simulink model "robot_segway_bloques"  (R2023b)
settings: Solver=ode15s  StartTime=0.0  StopTime=tiempo_final  MaxStep=1e-3  RelTol=1e-5  AbsTol=1e-7
values from neighbouring files (symbols this model uses):
  par = parametros_simulink(P, C)    [cargar_workspace.m]    (also in construir_robot_bloques.m = -R f   (manual sec. 7)'; simular_ode.m)
  Ts = se.Ts    [robot_controlador.m]    (also in simular_ode.m = P.sens.Ts; simular_slx.m = P.sens.Ts)
undefined symbols (not defined in the file or in its folder): angulo_servo_inicial, encoders_iniciales, estados_iniciales, inclinacion_inicial_est, medidas_iniciales, retardo_muestras, semilla
libraries: simulink x10
(part 1 of 2)
settings Model: Creator=calde  LastModifiedBy=calde

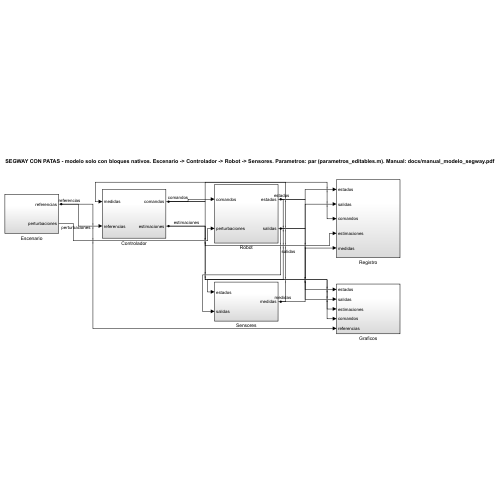
[thumbnail: Simulink's stored preview of the top-level diagram]
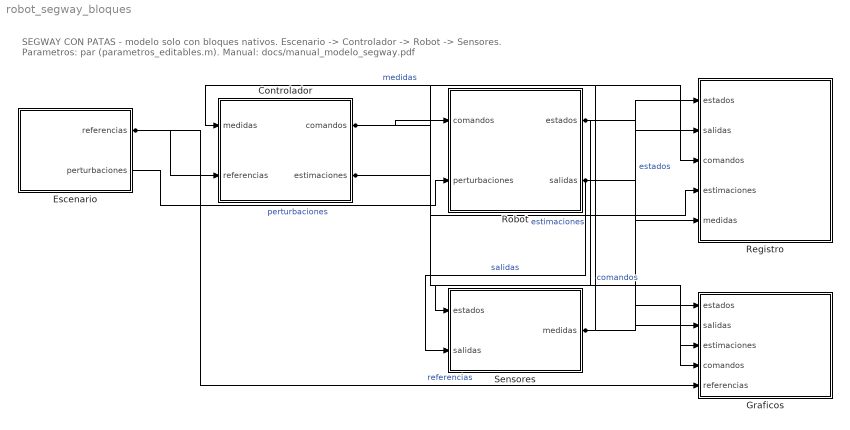
== system robot_segway_bloques ==
  note: SEGWAY CON PATAS - modelo solo con bloques nativos. Escenario -> Controlador -> Robot -> Sensores. Parametros: par (parametros_editables.m). Manual: docs/manual_modelo_segway.pdf
  Controlador : Subsystem
  Escenario : Subsystem
  Graficos : Subsystem
  Registro : Subsystem
  Robot : Subsystem
  Sensores : Subsystem
  wires:
  Escenario/1(referencias) -> Controlador/2(referencias), Graficos/5(referencias)  "referencias"
  Escenario/2(perturbaciones) -> Robot/2(perturbaciones)  "perturbaciones"
  Controlador/1(comandos) -> Robot/1(comandos), Registro/3(comandos), Graficos/4(comandos)  "comandos"
  Robot/1(estados) -> Sensores/1(estados), Registro/1(estados), Graficos/1(estados)  "estados"
  Robot/2(salidas) -> Sensores/2(salidas), Registro/2(salidas), Graficos/2(salidas)  "salidas"
  Sensores/1(medidas) -> Controlador/1(medidas), Registro/5(medidas)  "medidas"
  Controlador/2(estimaciones) -> Registro/4(estimaciones), Graficos/3(estimaciones)  "estimaciones"

== system robot_segway_bloques/Controlador ==
  note: CONTROL discreto a Ts: odometria -> filtro complementario -> LQR programado por l -> tension por motor ; consigna del servo con limite de velocidad
  medidas : Inport
  referencias : Inport  Port=2
  Consigna del servo : Subsystem
  Inclinacion (filtro complementario) : Subsystem
  LQR programado por largo de pata : Subsystem
  Odometria (encoders) : Subsystem
  Par de rueda a tension de motores : Subsystem
  comandos (3) : Mux  Inputs=3
  estimaciones (7) : Mux  Inputs=7
  separar medidas : Demux  Outputs=5
  separar referencias : Demux  Outputs=2
  comandos : Outport
  estimaciones : Outport  Port=2
  wires:
  medidas/1 -> separar medidas/1
  referencias/1 -> separar referencias/1
  separar medidas/4 -> Odometria (encoders)/1(encoder_izq)  "encoder_izq"
  separar medidas/5 -> Odometria (encoders)/2(encoder_der)  "encoder_der"
  separar medidas/1 -> Inclinacion (filtro complementario)/1(giroscopo), LQR programado por largo de pata/5(giroscopo)  "giroscopo"
  separar medidas/2 -> Inclinacion (filtro complementario)/2(acel_x)  "acel_x"
  separar medidas/3 -> Inclinacion (filtro complementario)/3(acel_y)  "acel_y"
  Odometria (encoders)/3(acel_est) -> Inclinacion (filtro complementario)/4(acel_base_est)  "acel_base_est"
  Odometria (encoders)/1(x_est) -> LQR programado por largo de pata/1(x_est), estimaciones (7)/2  "x_est"
  separar referencias/1 -> LQR programado por largo de pata/2(x_ref)  "x_ref"
  Inclinacion (filtro complementario)/1(inclinacion_est) -> LQR programado por largo de pata/3(inclinacion_est), estimaciones (7)/1  "inclinacion_est"
  Odometria (encoders)/2(dx_est) -> LQR programado por largo de pata/4(dx_est), estimaciones (7)/3  "dx_est"
  Consigna del servo/2(angulo_servo_anterior) -> LQR programado por largo de pata/6(angulo_servo_anterior)  "angulo_servo_anterior"
  LQR programado por largo de pata/1(par_rueda) -> Par de rueda a tension de motores/1(par_rueda), estimaciones (7)/5  "par_rueda_cmd"
  Odometria (encoders)/4(vel_ruedas_est) -> Par de rueda a tension de motores/2(vel_ruedas_est)  "vel_ruedas_est"
  separar referencias/2 -> Consigna del servo/1(l_ref)  "l_ref"
  Par de rueda a tension de motores/1(tension_izq) -> comandos (3)/1  "tension_izq"
  Par de rueda a tension de motores/2(tension_der) -> comandos (3)/2  "tension_der"
  Consigna del servo/1(angulo_servo_ref) -> comandos (3)/3  "angulo_servo_ref"
  LQR programado por largo de pata/2(largo_pata_est) -> estimaciones (7)/4  "largo_pata_est"
  Par de rueda a tension de motores/3(saturado) -> estimaciones (7)/6  "tension_saturada"
  Inclinacion (filtro complementario)/2(en_vuelo) -> estimaciones (7)/7  "en_vuelo"
  comandos (3)/1 -> comandos/1
  estimaciones (7)/1 -> estimaciones/1

== system robot_segway_bloques/Escenario ==
  note: Referencias y perturbaciones del escenario (escenarios_robot.m), desde el workspace
  "perturbaciones (F_x, M_p, pendiente, mu, F_escalon)" : FromWorkspace  VariableName=perturbaciones_ts  Interpolate=off  OutputAfterFinalValue=Holding final value
  "referencias (x_ref, l_ref)" : FromWorkspace  VariableName=referencias_ts  SampleTime=Ts  Interpolate=off  OutputAfterFinalValue=Holding final value
  referencias : Outport
  perturbaciones : Outport  Port=2
  wires:
  "referencias (x_ref, l_ref)"/1 -> referencias/1  "referencias"
  "perturbaciones (F_x, M_p, pendiente, mu, F_escalon)"/1 -> perturbaciones/1  "perturbaciones"

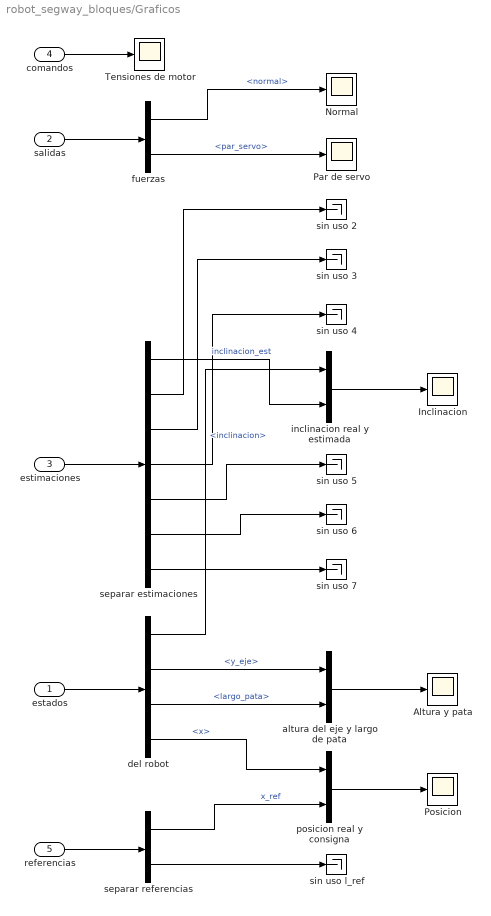
== system robot_segway_bloques/Graficos ==
  estados : Inport
  salidas : Inport  Port=2
  estimaciones : Inport  Port=3
  comandos : Inport  Port=4
  referencias : Inport  Port=5
  Altura y pata : Scope
  Inclinacion : Scope
  Normal : Scope
  Par de servo : Scope
  Posicion : Scope
  Tensiones de motor : Scope
  altura del eje y largo de pata : Mux  Inputs=2
  del robot : BusSelector  OutputSignals=inclinacion,y_eje,largo_pata,x
  fuerzas : BusSelector  OutputSignals=normal,par_servo
  inclinacion real y estimada : Mux  Inputs=2
  posicion real y consigna : Mux  Inputs=2
  separar estimaciones : Demux  Outputs=7
  separar referencias : Demux  Outputs=2
  sin uso {2..7} (6 alike) : Terminator
  sin uso l_ref : Terminator
  wires:
  separar estimaciones/1 -> inclinacion real y estimada/2  "inclinacion_est"
  fuerzas/2 -> Par de servo/1  "<par_servo>"
  comandos/1 -> Tensiones de motor/1
  separar referencias/2 -> sin uso l_ref/1
  salidas/1 -> fuerzas/1
  estimaciones/1 -> separar estimaciones/1
  fuerzas/1 -> Normal/1  "<normal>"
  referencias/1 -> separar referencias/1
  estados/1 -> del robot/1
  separar estimaciones/2 -> sin uso 2/1
  separar estimaciones/3 -> sin uso 3/1
  separar estimaciones/4 -> sin uso 4/1
  separar estimaciones/5 -> sin uso 5/1
  separar estimaciones/6 -> sin uso 6/1
  separar estimaciones/7 -> sin uso 7/1
  del robot/1 -> inclinacion real y estimada/1  "<inclinacion>"
  altura del eje y largo de pata/1 -> Altura y pata/1
  del robot/2 -> altura del eje y largo de pata/1  "<y_eje>"
  del robot/3 -> altura del eje y largo de pata/2  "<largo_pata>"
  del robot/4 -> posicion real y consigna/1  "<x>"
  separar referencias/1 -> posicion real y consigna/2  "x_ref"
  inclinacion real y estimada/1 -> Inclinacion/1
  posicion real y consigna/1 -> Posicion/1

== system robot_segway_bloques/Registro ==
  note: Se guardan en el workspace: estados, salidas, comandos, estimaciones, medidas (simular_slx los convierte en matrices)
  estados : Inport
  salidas : Inport  Port=2
  comandos : Inport  Port=3
  estimaciones : Inport  Port=4
  medidas : Inport  Port=5
  a workspace: comandos : ToWorkspace  VariableName=comandos  SaveFormat=Timeseries  SampleTime=-1
  a workspace: estados : ToWorkspace  VariableName=estados  SaveFormat=Timeseries  SampleTime=-1
  a workspace: estimaciones : ToWorkspace  VariableName=estimaciones  SaveFormat=Timeseries  SampleTime=-1
  a workspace: medidas : ToWorkspace  VariableName=medidas  SaveFormat=Timeseries  SampleTime=-1
  a workspace: salidas : ToWorkspace  VariableName=salidas  SaveFormat=Timeseries  SampleTime=-1
  wires:
  estimaciones/1 -> a workspace: estimaciones/1
  salidas/1 -> a workspace: salidas/1
  medidas/1 -> a workspace: medidas/1
  comandos/1 -> a workspace: comandos/1
  estados/1 -> a workspace: estados/1

== system robot_segway_bloques/Robot ==
  note: PLANTA: cada parte publica un bus con su nombre y los demas eligen lo que usan (Bus Selector). Estados y salidas en el mismo orden que robot_planta.m
  comandos : Inport
  perturbaciones : Inport  Port=2
  Bateria y puente H : Subsystem
  Contacto rueda-piso : Subsystem
  Cuerpo (Lagrange) : Subsystem
  Estados y salidas con nombre : Subsystem
  IMU (fuerza especifica) : Subsystem
  Motores y reductores : Subsystem
  Piso con escalones : Subsystem
  Ruedas : Subsystem
  Servo y pata : Subsystem
  bus comandos : BusCreator  Inputs=3
  bus perturbaciones : BusCreator  Inputs=5
  separar comandos : Demux  Outputs=3
  separar perturbaciones : Demux  Outputs=5
  estados : Outport
  salidas : Outport  Port=2
  wires:
  comandos/1 -> separar comandos/1
  separar comandos/1 -> bus comandos/1  "tension_izq"
  separar comandos/2 -> bus comandos/2  "tension_der"
  separar comandos/3 -> bus comandos/3  "angulo_servo_ref"
  perturbaciones/1 -> separar perturbaciones/1
  separar perturbaciones/1 -> bus perturbaciones/1  "F_x"
  separar perturbaciones/2 -> bus perturbaciones/2  "M_p"
  separar perturbaciones/3 -> bus perturbaciones/3  "pendiente"
  separar perturbaciones/4 -> bus perturbaciones/4  "mu"
  separar perturbaciones/5 -> bus perturbaciones/5  "F_escalon"
  bus comandos/1 -> Bateria y puente H/1(comandos), Servo y pata/1(comandos)  "comandos"
  bus perturbaciones/1 -> Contacto rueda-piso/4(perturbaciones), Cuerpo (Lagrange)/4(perturbaciones), IMU (fuerza especifica)/2(perturbaciones)  "perturbaciones"
  Bateria y puente H/1(bateria) -> Motores y reductores/1(bateria), Estados y salidas con nombre/5(bateria)  "bateria"
  Motores y reductores/1(motores) -> Bateria y puente H/2(motores), Ruedas/1(motores), Cuerpo (Lagrange)/2(motores), Estados y salidas con nombre/3(motores)  "motores"
  Ruedas/1(ruedas) -> Motores y reductores/2(ruedas), Contacto rueda-piso/2(ruedas), Estados y salidas con nombre/2(ruedas)  "ruedas"
  Piso con escalones/1(piso) -> Contacto rueda-piso/3(piso), Estados y salidas con nombre/7(piso)  "piso"
  Contacto rueda-piso/1(contacto) -> Ruedas/2(contacto), Cuerpo (Lagrange)/1(contacto), Estados y salidas con nombre/6(contacto)  "contacto"
  Servo y pata/1(pata) -> Cuerpo (Lagrange)/3(pata), Estados y salidas con nombre/4(pata)  "pata"
  Cuerpo (Lagrange)/1(cuerpo) -> Piso con escalones/1(cuerpo), Contacto rueda-piso/1(cuerpo), Servo y pata/2(cuerpo), IMU (fuerza especifica)/1(cuerpo), Estados y salidas con nombre/1(cuerpo)  "cuerpo"
  IMU (fuerza especifica)/1(imu) -> Estados y salidas con nombre/8(imu)  "imu"
  Estados y salidas con nombre/1(estados) -> estados/1  "estados"
  Estados y salidas con nombre/2(salidas) -> salidas/1  "salidas"

== system robot_segway_bloques/Sensores ==
  note: IMU y encoders muestreados a Ts: giroscopo con sesgo, ruido y saturacion ; acelerometro con ruido ; encoders en cuentas enteras ; retardo de retardo_muestras
  estados : Inport
  salidas : Inport  Port=2
  Acelerometro : Subsystem
  Encoders : Subsystem
  Giroscopio : Subsystem
  de la IMU : BusSelector  OutputSignals=imu_fx,imu_fy
  del robot : BusSelector  OutputSignals=d_inclinacion,ang_rueda_izq,ang_rueda_der
  medidas (5) : Mux  Inputs=5
  muestreo del giro : ZeroOrderHold  SampleTime=Ts
  muestreo f_x : ZeroOrderHold  SampleTime=Ts
  muestreo f_y : ZeroOrderHold  SampleTime=Ts
  muestreo rueda der : ZeroOrderHold  SampleTime=Ts
  muestreo rueda izq : ZeroOrderHold  SampleTime=Ts
  retardo del bus de sensores : Delay  DelayLength=retardo_muestras  InitialCondition=medidas_iniciales  SampleTime=Ts
  medidas : Outport
  wires:
  del robot/3 -> muestreo rueda der/1  "<ang_rueda_der>"
  Encoders/2(encoder_der) -> medidas (5)/5  "encoder_der"
  de la IMU/2 -> muestreo f_y/1  "<imu_fy>"
  salidas/1 -> de la IMU/1
  estados/1 -> del robot/1
  muestreo del giro/1 -> Giroscopio/1(vel_cabeceo)  "vel_cabeceo"
  del robot/2 -> muestreo rueda izq/1  "<ang_rueda_izq>"
  Acelerometro/2(acel_y) -> medidas (5)/3  "acel_y"
  de la IMU/1 -> muestreo f_x/1  "<imu_fx>"
  del robot/1 -> muestreo del giro/1  "<d_inclinacion>"
  muestreo f_x/1 -> Acelerometro/1(f_x)  "f_x"
  Encoders/1(encoder_izq) -> medidas (5)/4  "encoder_izq"
  muestreo f_y/1 -> Acelerometro/2(f_y)  "f_y"
  medidas (5)/1 -> retardo del bus de sensores/1  "medidas_sin_retardo"
  muestreo rueda izq/1 -> Encoders/1(ang_izq)  "ang_izq"
  muestreo rueda der/1 -> Encoders/2(ang_der)  "ang_der"
  Giroscopio/1(giroscopo) -> medidas (5)/1  "giroscopo"
  Acelerometro/1(acel_x) -> medidas (5)/2  "acel_x"
  retardo del bus de sensores/1 -> medidas/1  "medidas"

== system robot_segway_bloques/Controlador/Consigna del servo ==
  note: theta_ref = theta(l_ref) con limite de velocidad 0.8 w_vacio y acotada al rango del servo
  l_ref : Inport
  angulo objetivo theta(l_ref) : Lookup_n-D  NumberOfTableDimensions=1  BreakpointsForDimension1=par.pata.tabla_l  Table=par.pata.tabla_theta  InternalRulePriority=Speed  RndMeth=Simplest
  consigna anterior : UnitDelay  InitialCondition=angulo_servo_inicial  SampleTime=Ts  HasFrameUpgradeWarning=on
  largo dentro de la carrera : Saturate  UpperLimit=par.pata.l_max  LowerLimit=par.pata.l_min
  limitador de velocidad del servo : RateLimiter  RisingSlewLimit=0.8*par.servo.w_vacio  FallingSlewLimit=-(0.8*par.servo.w_vacio)  SampleTimeMode=inherited  InitialCondition=angulo_servo_inicial
  rango del servo : Saturate  UpperLimit=par.servo.theta_max  LowerLimit=par.servo.theta_min
  angulo_servo_ref : Outport
  angulo_servo_anterior : Outport  Port=2
  wires:
  consigna anterior/1 -> angulo_servo_anterior/1
  limitador de velocidad del servo/1 -> rango del servo/1
  l_ref/1 -> largo dentro de la carrera/1
  rango del servo/1 -> consigna anterior/1, angulo_servo_ref/1  "angulo_servo_ref"
  angulo objetivo theta(l_ref)/1 -> limitador de velocidad del servo/1  "angulo_objetivo"
  largo dentro de la carrera/1 -> angulo objetivo theta(l_ref)/1  "l_ref_acotado"

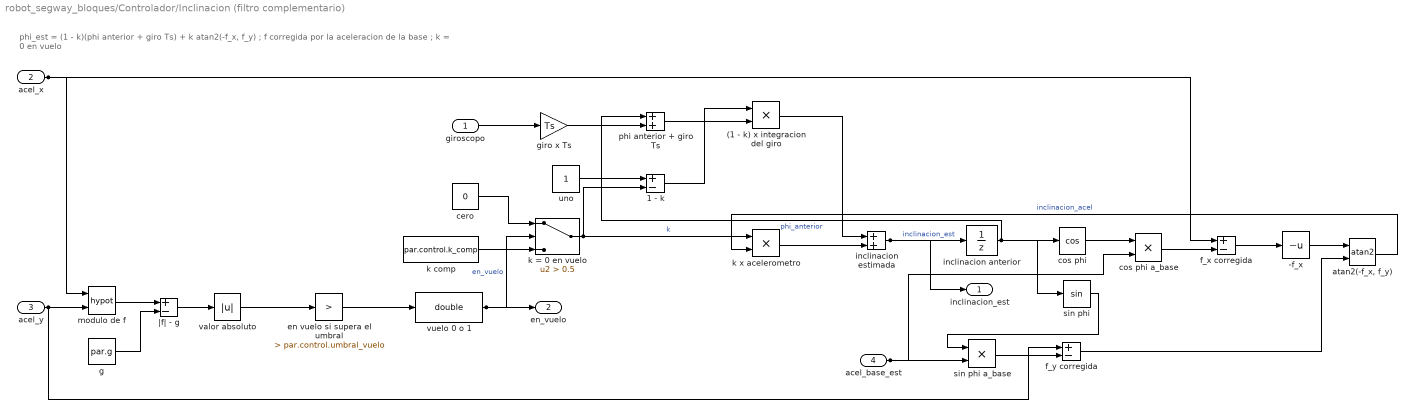
== system robot_segway_bloques/Controlador/Inclinacion (filtro complementario) ==
  note: phi_est = (1 - k)(phi anterior + giro Ts) + k atan2(-f_x, f_y) ; f corregida por la aceleracion de la base ; k = 0 en vuelo
  giroscopo : Inport
  acel_x : Inport  Port=2
  acel_y : Inport  Port=3
  acel_base_est : Inport  Port=4
  (1 - k) x integracion del giro : Product  Inputs=**
  -f_x : UnaryMinus
  1 - k : Sum  Inputs=+-
  "atan2(-f_x, f_y)" : Trigonometry  Operator=atan2
  cero : Constant  Value=0
  cos phi : Trigonometry  Operator=cos
  cos phi a_base : Product  Inputs=**
  en vuelo si supera el umbral : simulink/Logic and Bit Operations/Compare To Constant  relop=>  const=par.control.umbral_vuelo  OutDataTypeStr=boolean
  f_x corregida : Sum  Inputs=+-
  f_y corregida : Sum  Inputs=+-
  g : Constant  Value=par.g
  giro x Ts : Gain  Gain=Ts
  inclinacion anterior : UnitDelay  InitialCondition=inclinacion_inicial_est  SampleTime=Ts  HasFrameUpgradeWarning=on
  inclinacion estimada : Sum
  k = 0 en vuelo : Switch  Criteria=u2 > Threshold  Threshold=0.5  SaturateOnIntegerOverflow=off  InputSameDT=off
  k comp : Constant  Value=par.control.k_comp
  k x acelerometro : Product  Inputs=**
  modulo de f : Math  Operator=hypot
  phi anterior + giro Ts : Sum
  sin phi : Trigonometry
  sin phi a_base : Product  Inputs=**
  uno : Constant
  valor absoluto : Abs  SaturateOnIntegerOverflow=off
  vuelo 0 o 1 : DataTypeConversion  OutDataTypeStr=double  SaturateOnIntegerOverflow=off  RndMeth=Floor
  |f| - g : Sum  Inputs=+-
  inclinacion_est : Outport
  en_vuelo : Outport  Port=2
  wires:
  giroscopo/1 -> giro x Ts/1
  acel_y/1 -> f_y corregida/1, modulo de f/2
  acel_base_est/1 -> cos phi a_base/2, sin phi a_base/2
  (1 - k) x integracion del giro/1 -> inclinacion estimada/1
  acel_x/1 -> f_x corregida/1, modulo de f/1
  1 - k/1 -> (1 - k) x integracion del giro/1
  modulo de f/1 -> |f| - g/1
  g/1 -> |f| - g/2
  |f| - g/1 -> valor absoluto/1
  valor absoluto/1 -> en vuelo si supera el umbral/1
  en vuelo si supera el umbral/1 -> vuelo 0 o 1/1
  phi anterior + giro Ts/1 -> (1 - k) x integracion del giro/2
  cero/1 -> k = 0 en vuelo/1
  -f_x/1 -> "atan2(-f_x, f_y)"/1
  k comp/1 -> k = 0 en vuelo/3
  vuelo 0 o 1/1 -> en_vuelo/1, k = 0 en vuelo/2  "en_vuelo"
  giro x Ts/1 -> phi anterior + giro Ts/2
  uno/1 -> 1 - k/1
  k = 0 en vuelo/1 -> k x acelerometro/1, 1 - k/2  "k"
  k x acelerometro/1 -> inclinacion estimada/2
  "atan2(-f_x, f_y)"/1 -> k x acelerometro/2  "inclinacion_acel"
  inclinacion estimada/1 -> inclinacion anterior/1, inclinacion_est/1  "inclinacion_est"
  inclinacion anterior/1 -> phi anterior + giro Ts/1, sin phi/1, cos phi/1  "phi_anterior"
  cos phi a_base/1 -> f_x corregida/2
  sin phi a_base/1 -> f_y corregida/2
  sin phi/1 -> sin phi a_base/1
  cos phi/1 -> cos phi a_base/1
  f_y corregida/1 -> "atan2(-f_x, f_y)"/2
  f_x corregida/1 -> -f_x/1

== system robot_segway_bloques/Controlador/LQR programado por largo de pata ==
  note: par de rueda = -K(l) [x - x_ref ; phi ; dx ; dphi], K(l) = K1 + K2 l (manual sec. 10)
  x_est : Inport
  x_ref : Inport  Port=2
  inclinacion_est : Inport  Port=3
  dx_est : Inport  Port=4
  giroscopo : Inport  Port=5
  angulo_servo_anterior : Inport  Port=6
  K . error : DotProduct  OutDataTypeStr=Inherit: Inherit via internal rule
  K(l) = K1 + K2 l : Sum
  K1 : Constant  Value=par.control.K1(:)
  K2 x l : Gain  Gain=par.control.K2(:)
  dentro del rango del ajuste : Saturate  UpperLimit=par.control.l_max  LowerLimit=par.control.l_min
  error = [x - x_ref; phi; dx; dphi] : Mux
  error de posicion : Sum  Inputs=+-
  largo de pata segun angulo del servo : Lookup_n-D  NumberOfTableDimensions=1  BreakpointsForDimension1=par.pata.tabla_theta_inv  Table=par.pata.tabla_l_inv  InternalRulePriority=Speed  RndMeth=Simplest
  par = -K . error : UnaryMinus
  par_rueda : Outport
  largo_pata_est : Outport  Port=2
  wires:
  dx_est/1 -> error = [x - x_ref; phi; dx; dphi]/3
  angulo_servo_anterior/1 -> largo de pata segun angulo del servo/1
  largo de pata segun angulo del servo/1 -> dentro del rango del ajuste/1, largo_pata_est/1  "largo_pata_est"
  error de posicion/1 -> error = [x - x_ref; phi; dx; dphi]/1
  K2 x l/1 -> K(l) = K1 + K2 l/2
  dentro del rango del ajuste/1 -> K2 x l/1
  x_ref/1 -> error de posicion/2
  x_est/1 -> error de posicion/1
  K1/1 -> K(l) = K1 + K2 l/1
  giroscopo/1 -> error = [x - x_ref; phi; dx; dphi]/4
  inclinacion_est/1 -> error = [x - x_ref; phi; dx; dphi]/2
  K(l) = K1 + K2 l/1 -> K . error/1  "K"
  error = [x - x_ref; phi; dx; dphi]/1 -> K . error/2  "error"
  K . error/1 -> par = -K . error/1
  par = -K . error/1 -> par_rueda/1

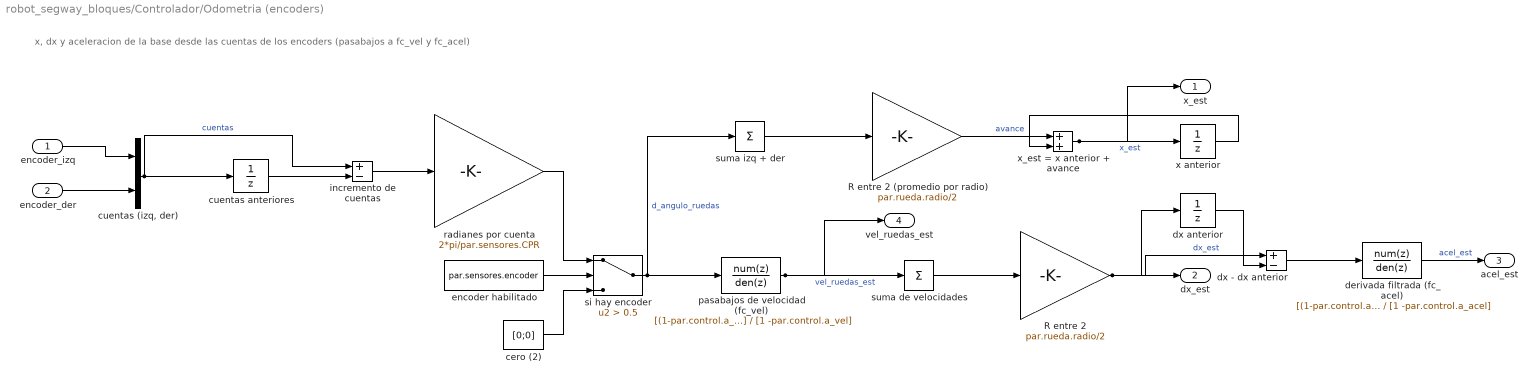
== system robot_segway_bloques/Controlador/Odometria (encoders) ==
  note: x, dx y aceleracion de la base desde las cuentas de los encoders (pasabajos a fc_vel y fc_acel)
  encoder_izq : Inport
  encoder_der : Inport  Port=2
  R entre 2 : Gain  Gain=par.rueda.radio/2
  R entre 2 (promedio por radio) : Gain  Gain=par.rueda.radio/2
  cero (2) : Constant  Value=[0;0]
  "cuentas (izq, der)" : Mux  Inputs=2
  cuentas anteriores : UnitDelay  InitialCondition=encoders_iniciales  SampleTime=Ts  HasFrameUpgradeWarning=on
  derivada filtrada (fc_acel) : DiscreteTransferFcn  Numerator=[(1-par.control.a_acel)/Ts 0]  Denominator=[1 -par.control.a_acel]  SampleTime=Ts
  dx - dx anterior : Sum  Inputs=+-
  dx anterior : UnitDelay  SampleTime=Ts  HasFrameUpgradeWarning=on
  encoder habilitado : Constant  Value=par.sensores.encoder
  incremento de cuentas : Sum  Inputs=+-
  pasabajos de velocidad (fc_vel) : DiscreteTransferFcn  Numerator=[(1-par.control.a_vel)/Ts 0]  Denominator=[1 -par.control.a_vel]  SampleTime=Ts
  radianes por cuenta : Gain  Gain=2*pi/par.sensores.CPR
  si hay encoder : Switch  Criteria=u2 > Threshold  Threshold=0.5  SaturateOnIntegerOverflow=off  InputSameDT=off
  suma de velocidades : Sum  Inputs=+
  suma izq + der : Sum  Inputs=+
  x anterior : UnitDelay  SampleTime=Ts  HasFrameUpgradeWarning=on
  x_est = x anterior + avance : Sum
  x_est : Outport
  dx_est : Outport  Port=2
  acel_est : Outport  Port=3
  vel_ruedas_est : Outport  Port=4
  wires:
  encoder_der/1 -> "cuentas (izq, der)"/2
  radianes por cuenta/1 -> si hay encoder/1
  R entre 2/1 -> dx - dx anterior/1, dx anterior/1, dx_est/1  "dx_est"
  encoder_izq/1 -> "cuentas (izq, der)"/1
  cero (2)/1 -> si hay encoder/3
  "cuentas (izq, der)"/1 -> incremento de cuentas/1, cuentas anteriores/1  "cuentas"
  cuentas anteriores/1 -> incremento de cuentas/2
  derivada filtrada (fc_acel)/1 -> acel_est/1  "acel_est"
  dx - dx anterior/1 -> derivada filtrada (fc_acel)/1
  incremento de cuentas/1 -> radianes por cuenta/1
  encoder habilitado/1 -> si hay encoder/2
  si hay encoder/1 -> pasabajos de velocidad (fc_vel)/1, suma izq + der/1  "d_angulo_ruedas"
  R entre 2 (promedio por radio)/1 -> x_est = x anterior + avance/1  "avance"
  suma izq + der/1 -> R entre 2 (promedio por radio)/1
  x_est = x anterior + avance/1 -> x anterior/1, x_est/1  "x_est"
  pasabajos de velocidad (fc_vel)/1 -> vel_ruedas_est/1, suma de velocidades/1  "vel_ruedas_est"
  dx anterior/1 -> dx - dx anterior/2
  suma de velocidades/1 -> R entre 2/1
  x anterior/1 -> x_est = x anterior + avance/2

== system robot_segway_bloques/Controlador/Par de rueda a tension de motores ==
  note: V = R (tau/2)/(Kt N eta) + Ke N w_est por motor, saturada a +-V_bat
  par_rueda : Inport
  vel_ruedas_est : Inport  Port=2
  R entre (2 Kt N eta) : Gain  Gain=par.motor.R/(2*par.motor.Kt*par.motor.relacion*par.motor.eta)
  alguna satura : Logic  Operator=OR  Inputs=1  AllPortsSameDT=off  OutDataTypeStr=boolean
  fcem Ke N w : Gain  Gain=par.motor.Ke*par.motor.relacion
  izq y der : Demux  Outputs=2
  limitar a la bateria : Saturate  UpperLimit=par.bateria.V  LowerLimit=-par.bateria.V
  saturado 0 o 1 : DataTypeConversion  OutDataTypeStr=double  SaturateOnIntegerOverflow=off  RndMeth=Floor
  supera V_bat : simulink/Logic and Bit Operations/Compare To Constant  relop=>  const=par.bateria.V  OutDataTypeStr=boolean
  "tension pedida (izq, der)" : Sum
  |V| : Abs  SaturateOnIntegerOverflow=off
  tension_izq : Outport
  tension_der : Outport  Port=2
  saturado : Outport  Port=3
  wires:
  par_rueda/1 -> R entre (2 Kt N eta)/1
  fcem Ke N w/1 -> "tension pedida (izq, der)"/2  "por_la_fcem"
  R entre (2 Kt N eta)/1 -> "tension pedida (izq, der)"/1  "por_el_par"
  vel_ruedas_est/1 -> fcem Ke N w/1
  limitar a la bateria/1 -> izq y der/1  "tension"
  "tension pedida (izq, der)"/1 -> |V|/1, limitar a la bateria/1  "tension_pedida"
  |V|/1 -> supera V_bat/1
  izq y der/1 -> tension_izq/1
  izq y der/2 -> tension_der/1
  supera V_bat/1 -> alguna satura/1
  alguna satura/1 -> saturado 0 o 1/1
  saturado 0 o 1/1 -> saturado/1

== system robot_segway_bloques/Robot/Bateria y puente H ==
  note: V_bus = max(V_bat - R_bat (|i_izq| + |i_der|), 0) ; V aplicada = sat(V pedida, -V_bus .. V_bus)
  comandos : Inport
  motores : Inport  Port=2
  -V_bus : UnaryMinus
  V_bat : Constant  Value=par.bateria.V
  V_bat - caida : Sum  Inputs=+-
  bus bateria : BusCreator  Inputs=3
  caida R_bat i : Gain  Gain=par.bateria.R
  cero : Constant  Value=0
  corriente total : Sum
  corrientes : BusSelector  OutputSignals=corriente_izq,corriente_der
  limitar der : simulink/Discontinuities/Saturation Dynamic  OutMin=[]  OutMax=[]  OutDataTypeStr=Inherit: Same as second input  OutDataType=fixdt(1, 16)  OutScaling=2^-10  DoSatur=off
  limitar izq : simulink/Discontinuities/Saturation Dynamic  OutMin=[]  OutMax=[]  OutDataTypeStr=Inherit: Same as second input  OutDataType=fixdt(1, 16)  OutScaling=2^-10  DoSatur=off
  no menor que 0 : MinMax  Function=max  Inputs=2
  tensiones pedidas : BusSelector  OutputSignals=tension_izq,tension_der
  |i der| : Abs  SaturateOnIntegerOverflow=off
  |i izq| : Abs  SaturateOnIntegerOverflow=off
  bateria : Outport
  wires:
  comandos/1 -> tensiones pedidas/1
  V_bat/1 -> V_bat - caida/1
  motores/1 -> corrientes/1
  corrientes/2 -> |i der|/1  "<corriente_der>"
  cero/1 -> no menor que 0/2
  corrientes/1 -> |i izq|/1  "<corriente_izq>"
  |i izq|/1 -> corriente total/1
  |i der|/1 -> corriente total/2
  no menor que 0/1 -> limitar izq/1, limitar der/1, bus bateria/1, -V_bus/1  "tension_bus"
  V_bat - caida/1 -> no menor que 0/1
  caida R_bat i/1 -> V_bat - caida/2  "caida"
  corriente total/1 -> caida R_bat i/1  "corriente_total"
  tensiones pedidas/1 -> limitar izq/2  "<tension_izq>"
  tensiones pedidas/2 -> limitar der/2  "<tension_der>"
  -V_bus/1 -> limitar der/3, limitar izq/3  "-tension_bus"
  limitar izq/1 -> bus bateria/2  "tension_aplicada_izq"
  limitar der/1 -> bus bateria/3  "tension_aplicada_der"
  bus bateria/1 -> bateria/1

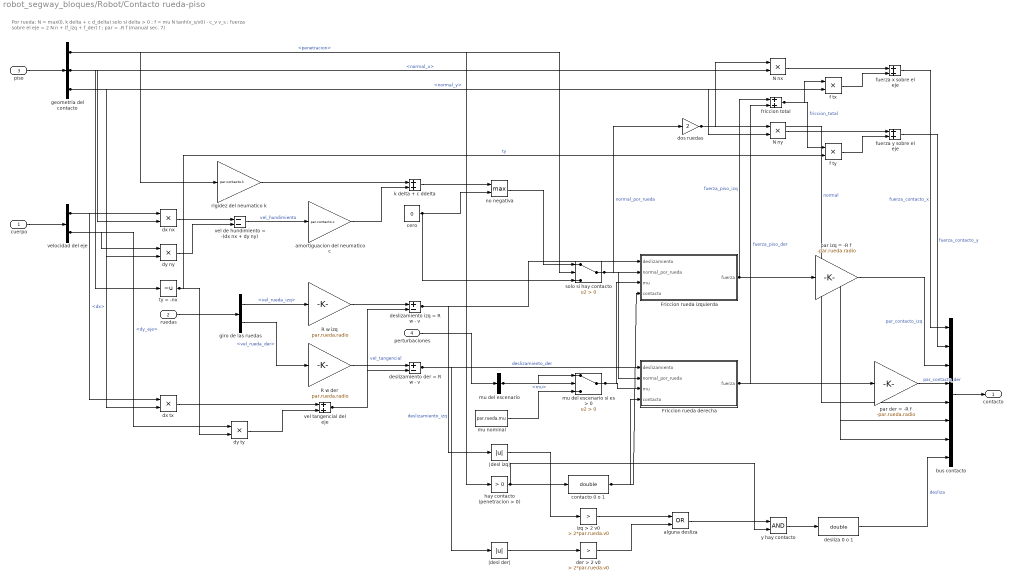
== system robot_segway_bloques/Robot/Contacto rueda-piso ==
  note: Por rueda: N = max(0, k delta + c d_delta) solo si delta > 0 ; f = mu N tanh(v_s/v0) - c_v v_s ; fuerza sobre el eje = 2 N n + (f_izq + f_der) t ; par = -R f (manual sec. 7)
  cuerpo : Inport
  ruedas : Inport  Port=2
  piso : Inport  Port=3
  perturbaciones : Inport  Port=4
  Friccion rueda derecha : Subsystem
  Friccion rueda izquierda : Subsystem
  N nx : Product  Inputs=**
  N ny : Product  Inputs=**
  R w der : Gain  Gain=par.rueda.radio
  R w izq : Gain  Gain=par.rueda.radio
  alguna desliza : Logic  Operator=OR  AllPortsSameDT=off  OutDataTypeStr=boolean
  amortiguacion del neumatico c : Gain  Gain=par.contacto.c
  bus contacto : BusCreator  Inputs=8
  cero : Constant  Value=0
  contacto 0 o 1 : DataTypeConversion  OutDataTypeStr=double  SaturateOnIntegerOverflow=off  RndMeth=Floor
  der > 2 v0 : simulink/Logic and Bit Operations/Compare To Constant  relop=>  const=2*par.rueda.v0  OutDataTypeStr=boolean
  desliza 0 o 1 : DataTypeConversion  OutDataTypeStr=double  SaturateOnIntegerOverflow=off  RndMeth=Floor
  deslizamiento der = R w - v : Sum  Inputs=+-
  deslizamiento izq = R w - v : Sum  Inputs=+-
  dos ruedas : Gain  Gain=2
  dx nx : Product  Inputs=**
  dx tx : Product  Inputs=**
  dy ny : Product  Inputs=**
  dy ty : Product  Inputs=**
  f tx : Product  Inputs=**
  f ty : Product  Inputs=**
  friccion total : Sum
  fuerza x sobre el eje : Sum
  fuerza y sobre el eje : Sum
  geometria del contacto : BusSelector  OutputSignals=penetracion,normal_x,normal_y
  giro de las ruedas : BusSelector  OutputSignals=vel_rueda_izq,vel_rueda_der
  hay contacto (penetracion > 0) : simulink/Logic and Bit Operations/Compare To Zero  relop=>  OutDataTypeStr=boolean
  izq > 2 v0 : simulink/Logic and Bit Operations/Compare To Constant  relop=>  const=2*par.rueda.v0  OutDataTypeStr=boolean
  k delta + c ddelta : Sum
  mu del escenario : BusSelector  OutputSignals=mu
  mu del escenario si es > 0 : Switch  Criteria=u2 > Threshold  SaturateOnIntegerOverflow=off  InputSameDT=off
  mu nominal : Constant  Value=par.rueda.mu
  no negativa : MinMax  Function=max  Inputs=2
  par der = -R f : Gain  Gain=-par.rueda.radio
  par izq = -R f : Gain  Gain=-par.rueda.radio
  rigidez del neumatico k : Gain  Gain=par.contacto.k
  solo si hay contacto : Switch  Criteria=u2 > Threshold  SaturateOnIntegerOverflow=off  InputSameDT=off
  ty = -nx : UnaryMinus
  vel de hundimiento = -(dx nx + dy ny) : Sum  Inputs=--
  vel tangencial del eje : Sum
  velocidad del eje : BusSelector  OutputSignals=dx,dy_eje
  y hay contacto : Logic  AllPortsSameDT=off  OutDataTypeStr=boolean
  |desl der| : Abs  SaturateOnIntegerOverflow=off
  |desl izq| : Abs  SaturateOnIntegerOverflow=off
  contacto : Outport
  wires:
  alguna desliza/1 -> y hay contacto/1
  no negativa/1 -> solo si hay contacto/1
  cuerpo/1 -> velocidad del eje/1
  mu del escenario si es > 0/1 -> Friccion rueda derecha/3(mu), Friccion rueda izquierda/3(mu)
  dx tx/1 -> vel tangencial del eje/1
  piso/1 -> geometria del contacto/1
  velocidad del eje/2 -> dy ty/1, dy ny/1  "<dy_eje>"
  geometria del contacto/3 -> f tx/2, N ny/2, dx tx/2, dy ny/2  "<normal_y>"
  velocidad del eje/1 -> dx nx/1, dx tx/1  "<dx>"
  desliza 0 o 1/1 -> bus contacto/8  "desliza"
  geometria del contacto/2 -> N nx/2, dx nx/2, ty = -nx/1  "<normal_x>"
  geometria del contacto/1 -> hay contacto (penetracion > 0)/1, rigidez del neumatico k/1, solo si hay contacto/2  "<penetracion>"
  solo si hay contacto/1 -> Friccion rueda izquierda/2(normal_por_rueda), Friccion rueda derecha/2(normal_por_rueda), dos ruedas/1  "normal_por_rueda"
  dx nx/1 -> vel de hundimiento = -(dx nx + dy ny)/1
  dy ny/1 -> vel de hundimiento = -(dx nx + dy ny)/2
  ty = -nx/1 -> f ty/2, dy ty/2  "ty"
  cero/1 -> solo si hay contacto/3, no negativa/2
  ruedas/1 -> giro de las ruedas/1
  vel de hundimiento = -(dx nx + dy ny)/1 -> amortiguacion del neumatico c/1  "vel_hundimiento"
  rigidez del neumatico k/1 -> k delta + c ddelta/1
  giro de las ruedas/1 -> R w izq/1  "<vel_rueda_izq>"
  giro de las ruedas/2 -> R w der/1  "<vel_rueda_der>"
  amortiguacion del neumatico c/1 -> k delta + c ddelta/2
  dy ty/1 -> vel tangencial del eje/2
  vel tangencial del eje/1 -> deslizamiento izq = R w - v/2, deslizamiento der = R w - v/2  "vel_tangencial"
  R w izq/1 -> deslizamiento izq = R w - v/1
  R w der/1 -> deslizamiento der = R w - v/1
  k delta + c ddelta/1 -> no negativa/1
  deslizamiento izq = R w - v/1 -> Friccion rueda izquierda/1(deslizamiento), |desl izq|/1  "deslizamiento_izq"
  perturbaciones/1 -> mu del escenario/1
  f tx/1 -> fuerza x sobre el eje/2
  deslizamiento der = R w - v/1 -> Friccion rueda derecha/1(deslizamiento), |desl der|/1  "deslizamiento_der"
  mu del escenario/1 -> mu del escenario si es > 0/1, mu del escenario si es > 0/2  "<mu>"
  Friccion rueda derecha/1(fuerza) -> par der = -R f/1, friccion total/2, bus contacto/7  "fuerza_piso_der"
  mu nominal/1 -> mu del escenario si es > 0/3
  izq > 2 v0/1 -> alguna desliza/1
  |desl izq|/1 -> izq > 2 v0/1
  |desl der|/1 -> der > 2 v0/1
  hay contacto (penetracion > 0)/1 -> y hay contacto/2, contacto 0 o 1/1
  contacto 0 o 1/1 -> Friccion rueda izquierda/4(contacto), Friccion rueda derecha/4(contacto)
  y hay contacto/1 -> desliza 0 o 1/1
  der > 2 v0/1 -> alguna desliza/2
  dos ruedas/1 -> bus contacto/5, N nx/1, N ny/1  "normal"
  Friccion rueda izquierda/1(fuerza) -> par izq = -R f/1, bus contacto/6, friccion total/1  "fuerza_piso_izq"
  N nx/1 -> fuerza x sobre el eje/1
  friccion total/1 -> f tx/1, f ty/1  "friccion_total"
  N ny/1 -> fuerza y sobre el eje/1
  f ty/1 -> fuerza y sobre el eje/2
  par izq = -R f/1 -> bus contacto/3  "par_contacto_izq"
  fuerza x sobre el eje/1 -> bus contacto/1  "fuerza_contacto_x"
  fuerza y sobre el eje/1 -> bus contacto/2  "fuerza_contacto_y"
  par der = -R f/1 -> bus contacto/4  "par_contacto_der"
  bus contacto/1 -> contacto/1

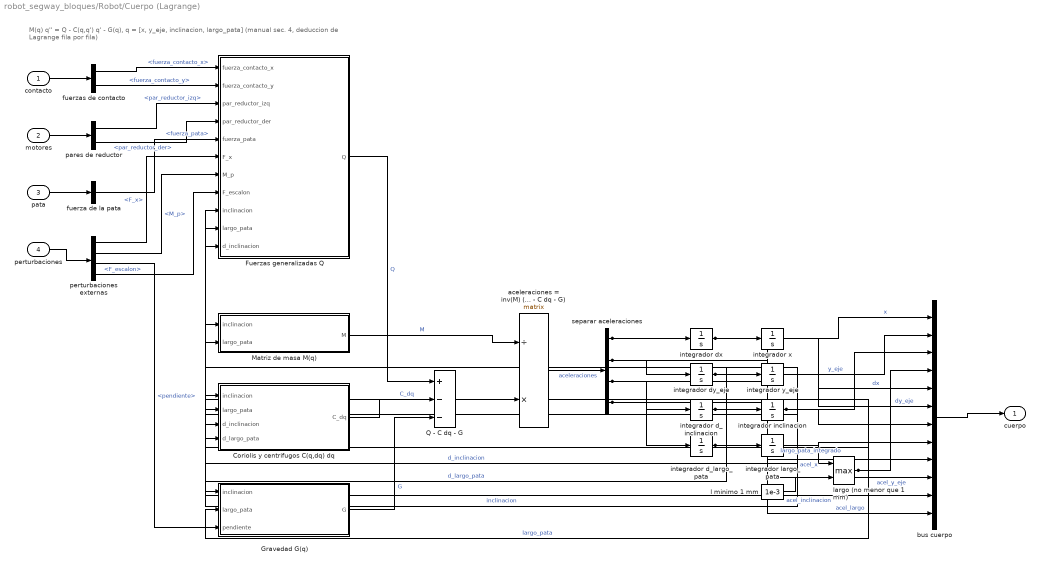
== system robot_segway_bloques/Robot/Cuerpo (Lagrange) ==
  note: M(q) q'' = Q - C(q,q') q' - G(q), q = [x, y_eje, inclinacion, largo_pata] (manual sec. 4, deduccion de Lagrange fila por fila)
  contacto : Inport
  motores : Inport  Port=2
  pata : Inport  Port=3
  perturbaciones : Inport  Port=4
  Coriolis y centrifugos C(q,dq) dq : Subsystem
  Fuerzas generalizadas Q : Subsystem
  Gravedad G(q) : Subsystem
  Matriz de masa M(q) : Subsystem
  Q - C dq - G : Sum  Inputs=+--
  aceleraciones = inv(M) (Q - C dq - G) : Product  Inputs=/*  Multiplication=Matrix(*)
  bus cuerpo : BusCreator  Inputs=12
  fuerza de la pata : BusSelector  OutputSignals=fuerza_pata
  fuerzas de contacto : BusSelector  OutputSignals=fuerza_contacto_x,fuerza_contacto_y
  integrador d_inclinacion : Integrator  InitialCondition=estados_iniciales(7)
  integrador d_largo_pata : Integrator  InitialCondition=estados_iniciales(8)
  integrador dx : Integrator  InitialCondition=estados_iniciales(5)
  integrador dy_eje : Integrator  InitialCondition=estados_iniciales(6)
  integrador inclinacion : Integrator  InitialCondition=estados_iniciales(3)
  integrador largo_pata : Integrator  InitialCondition=estados_iniciales(4)
  integrador x : Integrator  InitialCondition=estados_iniciales(1)
  integrador y_eje : Integrator  InitialCondition=estados_iniciales(2)
  l minimo 1 mm : Constant  Value=1e-3
  largo (no menor que 1 mm) : MinMax  Function=max  Inputs=2
  pares de reductor : BusSelector  OutputSignals=par_reductor_izq,par_reductor_der
  perturbaciones externas : BusSelector  OutputSignals=F_x,M_p,pendiente,F_escalon
  separar aceleraciones : Demux
  cuerpo : Outport
  wires:
  contacto/1 -> fuerzas de contacto/1
  motores/1 -> pares de reductor/1
  pata/1 -> fuerza de la pata/1
  perturbaciones/1 -> perturbaciones externas/1
  integrador dx/1 -> integrador x/1, bus cuerpo/5  "dx"
  integrador dy_eje/1 -> integrador y_eje/1, bus cuerpo/6  "dy_eje"
  integrador d_inclinacion/1 -> integrador inclinacion/1, Fuerzas generalizadas Q/11(d_inclinacion), Coriolis y centrifugos C(q,dq) dq/3(d_inclinacion), bus cuerpo/7  "d_inclinacion"
  integrador d_largo_pata/1 -> integrador largo_pata/1, Coriolis y centrifugos C(q,dq) dq/4(d_largo_pata), bus cuerpo/8  "d_largo_pata"
  integrador largo_pata/1 -> largo (no menor que 1 mm)/1  "largo_pata_integrado"
  l minimo 1 mm/1 -> largo (no menor que 1 mm)/2
  fuerzas de contacto/1 -> Fuerzas generalizadas Q/1(fuerza_contacto_x)  "<fuerza_contacto_x>"
  fuerzas de contacto/2 -> Fuerzas generalizadas Q/2(fuerza_contacto_y)  "<fuerza_contacto_y>"
  pares de reductor/1 -> Fuerzas generalizadas Q/3(par_reductor_izq)  "<par_reductor_izq>"
  pares de reductor/2 -> Fuerzas generalizadas Q/4(par_reductor_der)  "<par_reductor_der>"
  fuerza de la pata/1 -> Fuerzas generalizadas Q/5(fuerza_pata)  "<fuerza_pata>"
  perturbaciones externas/1 -> Fuerzas generalizadas Q/6(F_x)  "<F_x>"
  perturbaciones externas/2 -> Fuerzas generalizadas Q/7(M_p)  "<M_p>"
  perturbaciones externas/4 -> Fuerzas generalizadas Q/8(F_escalon)  "<F_escalon>"
  integrador inclinacion/1 -> Fuerzas generalizadas Q/9(inclinacion), Matriz de masa M(q)/1(inclinacion), Coriolis y centrifugos C(q,dq) dq/1(inclinacion), Gravedad G(q)/1(inclinacion), bus cuerpo/3  "inclinacion"
  largo (no menor que 1 mm)/1 -> Fuerzas generalizadas Q/10(largo_pata), Matriz de masa M(q)/2(largo_pata), Coriolis y centrifugos C(q,dq) dq/2(largo_pata), Gravedad G(q)/2(largo_pata), bus cuerpo/4  "largo_pata"
  perturbaciones externas/3 -> Gravedad G(q)/3(pendiente)  "<pendiente>"
  Fuerzas generalizadas Q/1(Q) -> Q - C dq - G/1  "Q"
  Coriolis y centrifugos C(q,dq) dq/1(C_dq) -> Q - C dq - G/2  "C_dq"
  Gravedad G(q)/1(G) -> Q - C dq - G/3  "G"
  Matriz de masa M(q)/1(M) -> aceleraciones = inv(M) (Q - C dq - G)/1  "M"
  Q - C dq - G/1 -> aceleraciones = inv(M) (Q - C dq - G)/2
  aceleraciones = inv(M) (Q - C dq - G)/1 -> separar aceleraciones/1  "aceleraciones"
  separar aceleraciones/1 -> integrador dx/1, bus cuerpo/9  "acel_x"
  separar aceleraciones/2 -> integrador dy_eje/1, bus cuerpo/10  "acel_y_eje"
  separar aceleraciones/3 -> integrador d_inclinacion/1, bus cuerpo/11  "acel_inclinacion"
  separar aceleraciones/4 -> integrador d_largo_pata/1, bus cuerpo/12  "acel_largo"
  integrador x/1 -> bus cuerpo/1  "x"
  integrador y_eje/1 -> bus cuerpo/2  "y_eje"
  bus cuerpo/1 -> cuerpo/1

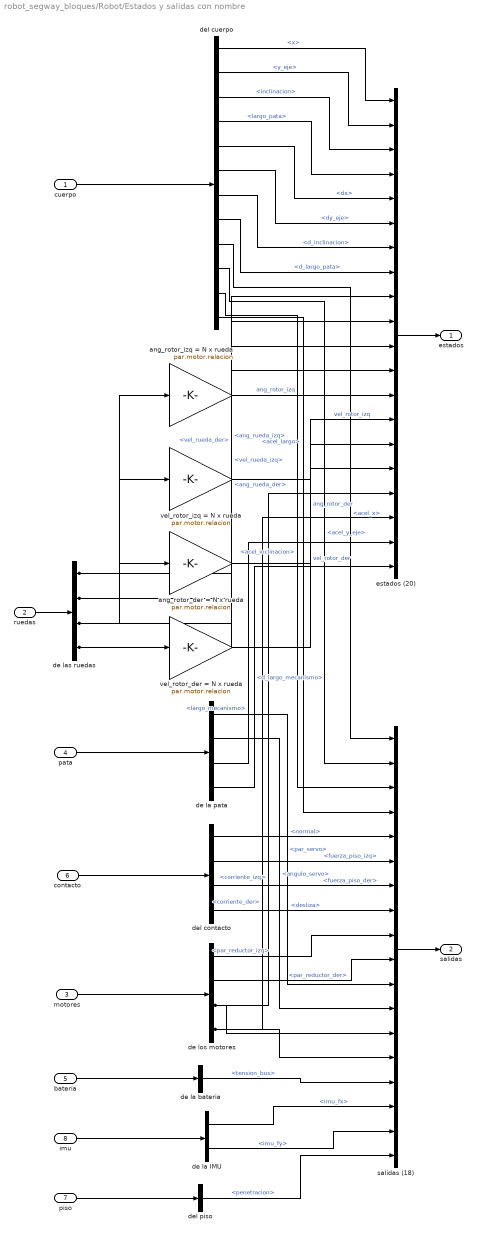
== system robot_segway_bloques/Robot/Estados y salidas con nombre ==
  cuerpo : Inport
  ruedas : Inport  Port=2
  motores : Inport  Port=3
  pata : Inport  Port=4
  bateria : Inport  Port=5
  contacto : Inport  Port=6
  piso : Inport  Port=7
  imu : Inport  Port=8
  ang_rotor_der = N x rueda : Gain  Gain=par.motor.relacion
  ang_rotor_izq = N x rueda : Gain  Gain=par.motor.relacion
  de la IMU : BusSelector  OutputSignals=imu_fx,imu_fy
  de la bateria : BusSelector  OutputSignals=tension_bus
  de la pata : BusSelector  OutputSignals=par_servo,angulo_servo,largo_mecanismo,d_largo_mecanismo
  de las ruedas : BusSelector  OutputSignals=ang_rueda_izq,vel_rueda_izq,ang_rueda_der,vel_rueda_der
  de los motores : BusSelector  OutputSignals=par_reductor_izq,par_reductor_der,corriente_izq,corriente_der
  del contacto : BusSelector  OutputSignals=normal,fuerza_piso_izq,fuerza_piso_der,desliza
  del cuerpo : BusSelector  OutputSignals=x,y_eje,inclinacion,largo_pata,dx,dy_eje,d_inclinacion,d_largo_pata,acel_x,acel_y_eje,acel_inclinacion,acel_largo
  del piso : BusSelector  OutputSignals=penetracion
  estados (20) : BusCreator  Inputs=20
  salidas (18) : BusCreator  Inputs=18
  vel_rotor_der = N x rueda : Gain  Gain=par.motor.relacion
  vel_rotor_izq = N x rueda : Gain  Gain=par.motor.relacion
  estados : Outport
  salidas : Outport  Port=2
  wires:
  de las ruedas/1 -> estados (20)/9, ang_rotor_izq = N x rueda/1  "<ang_rueda_izq>"
  contacto/1 -> del contacto/1
  del cuerpo/6 -> estados (20)/6  "<dy_eje>"
  pata/1 -> de la pata/1
  del cuerpo/2 -> estados (20)/2  "<y_eje>"
  imu/1 -> de la IMU/1
  ruedas/1 -> de las ruedas/1
  piso/1 -> del piso/1
  de las ruedas/3 -> estados (20)/11, ang_rotor_der = N x rueda/1  "<ang_rueda_der>"
  cuerpo/1 -> del cuerpo/1
  de las ruedas/2 -> estados (20)/10, vel_rotor_izq = N x rueda/1  "<vel_rueda_izq>"
  de las ruedas/4 -> estados (20)/12, vel_rotor_der = N x rueda/1  "<vel_rueda_der>"
  de los motores/2 -> salidas (18)/10  "<par_reductor_der>"
  motores/1 -> de los motores/1
  bateria/1 -> de la bateria/1
  del cuerpo/1 -> estados (20)/1  "<x>"
  del cuerpo/3 -> estados (20)/3  "<inclinacion>"
  del cuerpo/4 -> estados (20)/4  "<largo_pata>"
  del cuerpo/5 -> estados (20)/5  "<dx>"
  del cuerpo/7 -> estados (20)/7  "<d_inclinacion>"
  del cuerpo/8 -> estados (20)/8  "<d_largo_pata>"
  del cuerpo/9 -> salidas (18)/1  "<acel_x>"
  del cuerpo/10 -> salidas (18)/2  "<acel_y_eje>"
  del cuerpo/11 -> salidas (18)/3  "<acel_inclinacion>"
  del cuerpo/12 -> salidas (18)/4  "<acel_largo>"
  ang_rotor_izq = N x rueda/1 -> estados (20)/13  "ang_rotor_izq"
  vel_rotor_izq = N x rueda/1 -> estados (20)/14  "vel_rotor_izq"
  ang_rotor_der = N x rueda/1 -> estados (20)/15  "ang_rotor_der"
  vel_rotor_der = N x rueda/1 -> estados (20)/16  "vel_rotor_der"
  de la pata/1 -> salidas (18)/11  "<par_servo>"
  de la pata/2 -> salidas (18)/12  "<angulo_servo>"
  de la pata/3 -> estados (20)/19  "<largo_mecanismo>"
  de la pata/4 -> estados (20)/20  "<d_largo_mecanismo>"
  del contacto/1 -> salidas (18)/5  "<normal>"
  del contacto/2 -> salidas (18)/6  "<fuerza_piso_izq>"
  del contacto/3 -> salidas (18)/7  "<fuerza_piso_der>"
  del contacto/4 -> salidas (18)/8  "<desliza>"
  de los motores/1 -> salidas (18)/9  "<par_reductor_izq>"
  de los motores/3 -> estados (20)/17, salidas (18)/13  "<corriente_izq>"
  de los motores/4 -> estados (20)/18, salidas (18)/14  "<corriente_der>"
  de la bateria/1 -> salidas (18)/15  "<tension_bus>"
  de la IMU/1 -> salidas (18)/16  "<imu_fx>"
  de la IMU/2 -> salidas (18)/17  "<imu_fy>"
  del piso/1 -> salidas (18)/18  "<penetracion>"
  estados (20)/1 -> estados/1
  salidas (18)/1 -> salidas/1

== system robot_segway_bloques/Robot/IMU (fuerza especifica) ==
  note: Fuerza especifica en la IMU: aceleracion del CoM -> punto de la IMU (brazo d_i) -> menos gravedad -> rotada al marco cuerpo (manual sec. 9)
  cuerpo : Inport
  perturbaciones : Inport  Port=2
  Aceleracion del CoM : Subsystem
  Aceleracion en el punto de la IMU : Subsystem
  Fuerza especifica en marco cuerpo : Subsystem
  bus imu : BusCreator  Inputs=2
  movimiento del cuerpo : BusSelector  OutputSignals=inclinacion,largo_pata,d_inclinacion,d_largo_pata,acel_x,acel_y_eje,acel_inclinacion,acel_largo
  pendiente del piso : BusSelector  OutputSignals=pendiente
  imu : Outport
  wires:
  cuerpo/1 -> movimiento del cuerpo/1
  movimiento del cuerpo/7 -> Aceleracion en el punto de la IMU/5(acel_inclinacion), Aceleracion del CoM/3(acel_inclinacion)  "<acel_inclinacion>"
  movimiento del cuerpo/5 -> Aceleracion del CoM/1(acel_x_eje)  "<acel_x>"
  movimiento del cuerpo/3 -> Aceleracion en el punto de la IMU/4(d_inclinacion), Aceleracion del CoM/7(d_inclinacion)  "<d_inclinacion>"
  movimiento del cuerpo/1 -> Fuerza especifica en marco cuerpo/3(inclinacion), Aceleracion en el punto de la IMU/3(inclinacion), Aceleracion del CoM/5(inclinacion)  "<inclinacion>"
  movimiento del cuerpo/6 -> Aceleracion del CoM/2(acel_y_eje)  "<acel_y_eje>"
  movimiento del cuerpo/4 -> Aceleracion del CoM/8(d_largo_pata)  "<d_largo_pata>"
  pendiente del piso/1 -> Fuerza especifica en marco cuerpo/4(pendiente)  "<pendiente>"
  movimiento del cuerpo/2 -> Aceleracion del CoM/6(largo_pata)  "<largo_pata>"
  movimiento del cuerpo/8 -> Aceleracion del CoM/4(acel_largo)  "<acel_largo>"
  Aceleracion del CoM/1(a_x) -> Aceleracion en el punto de la IMU/1(a_com_x)  "acel_com_x"
  Aceleracion del CoM/2(a_y) -> Aceleracion en el punto de la IMU/2(a_com_y)  "acel_com_y"
  perturbaciones/1 -> pendiente del piso/1
  Aceleracion en el punto de la IMU/1(a_imu_x) -> Fuerza especifica en marco cuerpo/1(a_imu_x)  "acel_imu_x"
  Aceleracion en el punto de la IMU/2(a_imu_y) -> Fuerza especifica en marco cuerpo/2(a_imu_y)  "acel_imu_y"
  Fuerza especifica en marco cuerpo/1(fb_x) -> bus imu/1  "imu_fx"
  Fuerza especifica en marco cuerpo/2(fb_y) -> bus imu/2  "imu_fy"
  bus imu/1 -> imu/1

== system robot_segway_bloques/Robot/Motores y reductores ==
  note: Motor DC + reductor rigido (manual sec. 6): L di/dt = V - R i - Ke N w_rueda ; par_reductor = N (Kt i - tau_c tanh(w/0.5) - b w)
  bateria : Inport
  ruedas : Inport  Port=2
  Motor y reductor derecho : Subsystem
  Motor y reductor izquierdo : Subsystem
  bus motores : BusCreator  Inputs=4
  tensiones aplicadas : BusSelector  OutputSignals=tension_aplicada_izq,tension_aplicada_der
  velocidades de rueda : BusSelector  OutputSignals=vel_rueda_izq,vel_rueda_der
  motores : Outport
  wires:
  Motor y reductor izquierdo/2(corriente) -> bus motores/3  "corriente_izq"
  Motor y reductor izquierdo/1(par_reductor) -> bus motores/1  "par_reductor_izq"
  Motor y reductor derecho/2(corriente) -> bus motores/4  "corriente_der"
  bateria/1 -> tensiones aplicadas/1
  velocidades de rueda/2 -> Motor y reductor derecho/2(vel_rueda)  "<vel_rueda_der>"
  ruedas/1 -> velocidades de rueda/1
  velocidades de rueda/1 -> Motor y reductor izquierdo/2(vel_rueda)  "<vel_rueda_izq>"
  tensiones aplicadas/2 -> Motor y reductor derecho/1(tension)  "<tension_aplicada_der>"
  tensiones aplicadas/1 -> Motor y reductor izquierdo/1(tension)  "<tension_aplicada_izq>"
  Motor y reductor derecho/1(par_reductor) -> bus motores/2  "par_reductor_der"
  bus motores/1 -> motores/1

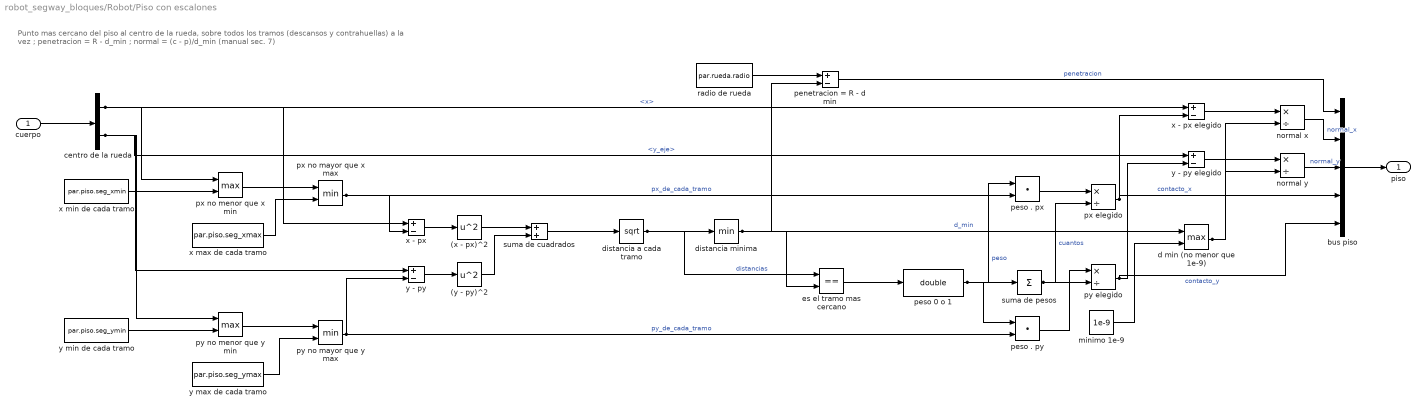
== system robot_segway_bloques/Robot/Piso con escalones ==
  note: Punto mas cercano del piso al centro de la rueda, sobre todos los tramos (descansos y contrahuellas) a la vez ; penetracion = R - d_min ; normal = (c - p)/d_min (manual sec. 7)
  cuerpo : Inport
  (x - px)^2 : Math  Operator=square
  (y - py)^2 : Math  Operator=square
  bus piso : BusCreator  Inputs=5
  centro de la rueda : BusSelector  OutputSignals=x,y_eje
  d min (no menor que 1e-9) : MinMax  Function=max  Inputs=2
  distancia a cada tramo : Sqrt
  distancia minima : MinMax
  es el tramo mas cercano : RelationalOperator  Operator===  OutDataTypeStr=boolean  RndMeth=Simplest  InputSameDT=off
  minimo 1e-9 : Constant  Value=1e-9
  normal x : Product  Inputs=*/
  normal y : Product  Inputs=*/
  penetracion = R - d min : Sum  Inputs=+-
  peso . px : DotProduct  OutDataTypeStr=Inherit: Inherit via internal rule
  peso . py : DotProduct  OutDataTypeStr=Inherit: Inherit via internal rule
  peso 0 o 1 : DataTypeConversion  OutDataTypeStr=double  SaturateOnIntegerOverflow=off  RndMeth=Floor
  px elegido : Product  Inputs=*/
  px no mayor que x max : MinMax  Inputs=2
  px no menor que x min : MinMax  Function=max  Inputs=2
  py elegido : Product  Inputs=*/
  py no mayor que y max : MinMax  Inputs=2
  py no menor que y min : MinMax  Function=max  Inputs=2
  radio de rueda : Constant  Value=par.rueda.radio
  suma de cuadrados : Sum
  suma de pesos : Sum  Inputs=+
  x - px : Sum  Inputs=+-
  x - px elegido : Sum  Inputs=+-
  x max de cada tramo : Constant  Value=par.piso.seg_xmax
  x min de cada tramo : Constant  Value=par.piso.seg_xmin
  y - py : Sum  Inputs=+-
  y - py elegido : Sum  Inputs=+-
  y max de cada tramo : Constant  Value=par.piso.seg_ymax
  y min de cada tramo : Constant  Value=par.piso.seg_ymin
  piso : Outport
  wires:
  py no menor que y min/1 -> py no mayor que y max/1
  es el tramo mas cercano/1 -> peso 0 o 1/1
  suma de cuadrados/1 -> distancia a cada tramo/1
  cuerpo/1 -> centro de la rueda/1
  centro de la rueda/2 -> y - py/1, y - py elegido/1, py no menor que y min/1  "<y_eje>"
  px no menor que x min/1 -> px no mayor que x max/1
  centro de la rueda/1 -> x - px elegido/1, x - px/1, px no menor que x min/1  "<x>"
  y min de cada tramo/1 -> py no menor que y min/2
  x min de cada tramo/1 -> px no menor que x min/2
  x max de cada tramo/1 -> px no mayor que x max/2
  y max de cada tramo/1 -> py no mayor que y max/2
  px no mayor que x max/1 -> peso . px/2, x - px/2  "px_de_cada_tramo"
  py no mayor que y max/1 -> peso . py/2, y - py/2  "py_de_cada_tramo"
  x - px/1 -> (x - px)^2/1
  y - py/1 -> (y - py)^2/1
  (x - px)^2/1 -> suma de cuadrados/1
  (y - py)^2/1 -> suma de cuadrados/2
  peso 0 o 1/1 -> peso . px/1, peso . py/1, suma de pesos/1  "peso"
  distancia a cada tramo/1 -> es el tramo mas cercano/1, distancia minima/1  "distancias"
  radio de rueda/1 -> penetracion = R - d min/1
  distancia minima/1 -> d min (no menor que 1e-9)/1, es el tramo mas cercano/2, penetracion = R - d min/2  "d_min"
  penetracion = R - d min/1 -> bus piso/1  "penetracion"
  peso . px/1 -> px elegido/1
  py elegido/1 -> bus piso/5, y - py elegido/2  "contacto_y"
  suma de pesos/1 -> px elegido/2, py elegido/2  "cuantos"
  peso . py/1 -> py elegido/1
  px elegido/1 -> x - px elegido/2, bus piso/4  "contacto_x"
  minimo 1e-9/1 -> d min (no menor que 1e-9)/2
  x - px elegido/1 -> normal x/1
  y - py elegido/1 -> normal y/1
  d min (no menor que 1e-9)/1 -> normal x/2, normal y/2
  normal x/1 -> bus piso/2  "normal_x"
  normal y/1 -> bus piso/3  "normal_y"
  bus piso/1 -> piso/1

== system robot_segway_bloques/Robot/Ruedas ==
  note: (J_rueda + N^2 J_rotor) dw/dt = par_reductor + par_contacto - b_w w (manual sec. 6: inercia reflejada del rotor)
  motores : Inport
  contacto : Inport  Port=2
  Rueda derecha : Subsystem
  Rueda izquierda : Subsystem
  bus ruedas : BusCreator  Inputs=4
  pares de contacto : BusSelector  OutputSignals=par_contacto_izq,par_contacto_der
  pares de reductor : BusSelector  OutputSignals=par_reductor_izq,par_reductor_der
  ruedas : Outport
  wires:
  bus ruedas/1 -> ruedas/1
  contacto/1 -> pares de contacto/1
  motores/1 -> pares de reductor/1
  pares de contacto/2 -> Rueda derecha/2(par_contacto)  "<par_contacto_der>"
  pares de contacto/1 -> Rueda izquierda/2(par_contacto)  "<par_contacto_izq>"
  pares de reductor/2 -> Rueda derecha/1(par_reductor)  "<par_reductor_der>"
  pares de reductor/1 -> Rueda izquierda/1(par_reductor)  "<par_reductor_izq>"
  Rueda izquierda/2(vel_rueda) -> bus ruedas/2  "vel_rueda_izq"
  Rueda izquierda/1(ang_rueda) -> bus ruedas/1  "ang_rueda_izq"
  Rueda derecha/1(ang_rueda) -> bus ruedas/3  "ang_rueda_der"
  Rueda derecha/2(vel_rueda) -> bus ruedas/4  "vel_rueda_der"
